simulink model "BD_PAR_AUTO_base_model"  (Simulink 10.3)
settings: Solver=ode1  StartTime=0.0  StopTime=max(cyc_mph(:,1))  FixedStep=1  MaxStep=1  RelTol=1e-3  AbsTol=1e-3
undefined symbols (not defined in the file): acc_dcdc_eff, acc_elec_eff, acc_elec_pwr, acc_mech_eff, acc_mech_pwr, acc_mech_trq, air_cp, amb_tmp, cs_charge_deplete_bool, cs_charge_trq, cs_electric_decel_spd, cs_electric_launch_spd_hi, cs_electric_launch_spd_lo, cs_hi_soc, cs_lo_soc, cs_min_trq_frac, cs_off_trq_frac, cyc_avg_time, cyc_cargo_mass, cyc_elevation_init, cyc_filter_bool, cyc_grade, cyc_mph, enable_sim_stop_distance, enable_sim_stop_max_spd, enable_sim_stop_speed, enable_sim_stop_time, enable_stop, enable_stop_fc, ess_cap_scale, ess_coulombic_eff, ess_init_soc, ess_max_ah_cap, ess_max_volts, ess_min_volts, ess_mod_airflow, ess_mod_cp, ess_mod_init_tmp, ess_module_mass, ess_module_num, ess_on, ess_r_chg, ess_r_dis, ess_res_scale_coef, ess_res_scale_fun, ess_set_tmp, ess_soc, ess_th_calc, ess_th_res_off, ess_th_res_on, ess_tmp, ess_voc, ex_calc, ex_cat_co_frac, ex_cat_ext_cp, ex_cat_ext_emisv, ex_cat_ext_init_tmp, ex_cat_ext_mass, ex_cat_ext_sarea, ex_cat_hc_frac ... (+168)
(part 2 of 15)

== system BD_PAR_AUTO_base_model/hydraulic torque converter for  parallel hybrid <htc> ==
  "req'd output trq and spd (Nm), (rad/s)" : Inport
  "trq and spd available at input (Nm), (rad/s)" : Inport  Port=2
  ">0 " : Saturate  UpperLimit=inf  LowerLimit=0
  >0. : Saturate  UpperLimit=inf  LowerLimit=0
  Block NOTES : Subsystem
      mask Display: disp('Block\nNOTES')
  Constant : Constant  Value=0
  Demux2 : Demux  Outputs=2
  Demux3 : Demux  Outputs=2
  Mux1 : Mux  Inputs=2
  Mux3 : Mux  Inputs=2
  Mux4 : Mux  Inputs=2
  SR : Subsystem
  "T, shifting" : Subsystem
  TR : Subsystem
  Tin= Tout,req/TR : Product  Inputs=/*  SaturateOnIntegerOverflow=on
  To Workspace : ToWorkspace  VariableName=htc_trq_in_r  SampleTime=-1
  To Workspace1 : ToWorkspace  VariableName=htc_spd_in_r  SampleTime=-1
  To Workspace10 : ToWorkspace  VariableName=htc_trq_inertia  SampleTime=-1
  To Workspace2 : ToWorkspace  VariableName=htc_trq_out_r  SampleTime=-1
  To Workspace3 : ToWorkspace  VariableName=htc_spd_out_r  SampleTime=-1
  To Workspace4 : ToWorkspace  VariableName=htc_trq_in_a  SampleTime=-1
  To Workspace5 : ToWorkspace  VariableName=htc_spd_in_a  SampleTime=-1
  To Workspace6 : ToWorkspace  VariableName=htc_trq_out_a  SampleTime=-1
  To Workspace7 : ToWorkspace  VariableName=htc_spd_out_a  SampleTime=-1
  To Workspace8 : ToWorkspace  VariableName=htc_sr_hist  SampleTime=-1
  To Workspace9 : ToWorkspace  VariableName=htc_tr_hist  SampleTime=-1
  Tout= Tin*TR : Product  Inputs=**  SaturateOnIntegerOverflow=on
  Tout_a =  Tout- Tinertia : Sum  Inputs=-+  SaturateOnIntegerOverflow=on
  "Treq, in =  Tin+ Tinertia" : Sum  SaturateOnIntegerOverflow=on
  effect of inertia (Nm) : Subsystem
  "shifting, ignore inertia torque in request" : Switch  Threshold=eps
  win= wout/SR : Product  Inputs=*/  SaturateOnIntegerOverflow=on
  wout= win*SR : Product  Inputs=**  SaturateOnIntegerOverflow=on
  "req'd input trq and spd (Nm), (rad/s)" : Outport  InitialOutput=0
  "trq and spd available at output (Nm), (rad/s)" : Outport  Port=2  InitialOutput=0
  wires:
  [shifting] -> "shifting, ignore inertia torque in request"/2
  >0./1 -> Mux3/2, To Workspace7/1
  wout= win*SR/1 -> >0./1
  Demux3/1 -> To Workspace4/1, Tout= Tin*TR/2
  "trq and spd available at input (Nm), (rad/s)"/1 -> Demux3/1
  Tout= Tin*TR/1 -> Tout_a =  Tout- Tinertia/2
  Mux3/1 -> "trq and spd available at output (Nm), (rad/s)"/1
  win= wout/SR/1 -> ">0 "/1
  "T, shifting"/1(T req) -> Mux4/1, Tin= Tout,req/TR/2, To Workspace2/1
  Demux2/1 -> "T, shifting"/3(Req'd output trq)
  Demux3/2 -> To Workspace5/1, wout= win*SR/2, SR/2(w in), "T, shifting"/4(htc_spd_in_a)
  Mux4/1 -> SR/1(T,w req out)
  SR/1(SR) -> win= wout/SR/2, wout= win*SR/1, To Workspace8/1, "T, shifting"/5(SR), TR/1(SR)
  Tout_a =  Tout- Tinertia/1 -> Mux3/1, To Workspace6/1
  Demux2/2 -> Mux4/2, win= wout/SR/1, effect of inertia (Nm)/1(turbine/output speed (rad/s)), To Workspace3/1
  ">0 "/1 -> To Workspace1/1, Mux1/2
  Constant/1 -> "shifting, ignore inertia torque in request"/1
  effect of inertia (Nm)/1(inertia torque (Nm)) -> Tout_a =  Tout- Tinertia/1, To Workspace10/1, "shifting, ignore inertia torque in request"/3
  TR/1(TR) -> Tout= Tin*TR/1, To Workspace9/1, Tin= Tout,req/TR/1, "T, shifting"/1(TR)
  SR/2(coasting) -> TR/2(coasting)
  Mux1/1 -> "req'd input trq and spd (Nm), (rad/s)"/1
  "Treq, in =  Tin+ Tinertia"/1 -> Mux1/1, To Workspace/1, "T, shifting"/2(Req'd  input trq)
  "shifting, ignore inertia torque in request"/1 -> "Treq, in =  Tin+ Tinertia"/2
  Tin= Tout,req/TR/1 -> "Treq, in =  Tin+ Tinertia"/1
  "req'd output trq and spd (Nm), (rad/s)"/1 -> Demux2/1

== system BD_PAR_AUTO_base_model/mechanical accessory loads <acc> ==
  note: from <fc>
  note: from <fc>
  note: torque req
  note: speed req
  note: aux spd req
  note: torque achieved
  note: speed achieved
  note: aux spd achieved
  note: from <vc>
  In1 : Inport
  In2 : Inport  Port=2
  Constant : Constant  Value=eps
  Demux : Demux  Outputs=2
      settings: DisplayOption=none
  Demux1 : Demux  Outputs=2
      settings: DisplayOption=none
  Logical Operator : Logic
  Mechanical Accessory Loads v2 <acc> : Subsystem  mask{load_on=not(ess_on)*1, acc_max_spd=inf, acc_min_spd=vc_idle_spd+eps, ic_mech_trq=0, ic_mech_pwr=0}
      mask prompts: load_on "Electrical Load Status: 1 on; 0 off"; acc_max_spd "maximum shaft speed for aux. (rad/s)"; acc_min_spd "minimum shaft speed for aux. (rad/s)"; ic_mech_trq "Initial Mechanical Torque of the Accessory Loads (Nm)"; ic_mech_pwr "Initial Mechanical Auxiliary Load Power (W)"
      mask Display: image(imread('bdi_acc_pic.bmp'))
  Mux : Mux  Inputs=3
  Mux1 : Mux  Inputs=3
  Relational Operator : RelationalOperator  Operator=>  RndMeth=Nearest  InputSameDT=on
  Out1 : Outport
  Out2 : Outport  Port=2
  wires:
  [signal_one] -> Mechanical Accessory Loads v2 <acc>/1("requested shaft T and w, out to the driveline  (Nm ; rad/s; rad/s)")
  Mechanical Accessory Loads v2 <acc>/1("requested shaft and belt T and w, in from the prime mover (Nm ; rad/s)") -> Out1/1
  Mechanical Accessory Loads v2 <acc>/2("achieved shaft T and w, out to the driveline (Nm ; rad/s)") -> Out2/1
  [signal_two] -> Mechanical Accessory Loads v2 <acc>/2("achieved shaft and belt T and w, in from the prime mover (Nm ; rad/s)")
  [acc_on] -> Mechanical Accessory Loads v2 <acc>/3(accessory on/off)
  Mux/1 -> [signal_one]
  In1/1 -> Demux/1
  Demux/1 -> Mux/1
  Demux/2 -> Mux/2
  [fc_spd_est] -> Mux/3
  Mux1/1 -> [signal_two]
  In2/1 -> Demux1/1
  Demux1/1 -> Mux1/1
  Demux1/2 -> Mux1/2
  [fc_spd_est] -> Mux1/3
  [fc_spd_est] -> Relational Operator/1
  Constant/1 -> Relational Operator/2
  [engine_on] -> Logical Operator/1
  Relational Operator/1 -> Logical Operator/2
  Logical Operator/1 -> [acc_on]

== system BD_PAR_AUTO_base_model/motor/ controller <mc> par ==
  "torque and speed  req'd at rotor (Nm), (rad/s)" : Inport
  available motor input power (W) : Inport  Port=2
  Block NOTES : Subsystem
      mask Display: disp('Block\nNOTES')
  Constant : Constant  Value=mc_eff_scale
  Demux : Demux  Outputs=2
  Fcn : Fcn  Expr=u[3]-u[1]*u[2]
  Mux2 : Mux  Inputs=2
  Mux3 : Mux  Inputs=3
  N-m drive torque per W input : Subsystem
  Product : Product  SaturateOnIntegerOverflow=on
  Product1 : Product  Inputs=*/  SaturateOnIntegerOverflow=on
  Saturation : Saturate  UpperLimit=max(mc_map_spd)*mc_spd_scale  LowerLimit=0
  Sum : Sum  SaturateOnIntegerOverflow=on
  Sum1 : Sum  Inputs=-+  SaturateOnIntegerOverflow=on
  Switch : Switch
  To WS1 : ToWorkspace  VariableName=mc_pwr_loss
      settings: MaxDataPoints=50000
  To WS2 : ToWorkspace  VariableName=mc_tmp
      settings: MaxDataPoints=50000
  To WS4 : ToWorkspace  VariableName=mc_clt_th_pwr
      settings: MaxDataPoints=50000
  To Workspace10 : ToWorkspace  VariableName=mc_ni_trq_out_a  SampleTime=-1
  To Workspace4 : ToWorkspace  VariableName=mc_trq_out_r  SampleTime=-1
  To Workspace5 : ToWorkspace  VariableName=mc_spd_out_r  SampleTime=-1
  To Workspace8 : ToWorkspace  VariableName=mc_pwr_in_a  SampleTime=-1
  To Workspace9 : ToWorkspace  VariableName=mc_pwr_in_r  SampleTime=-1
  do ex calcs? : Constant  Value=mc_th_calc
  documentation10 : Subsystem
      settings: OpenFcn=web(['file:\\\' which('motor_controller.htm')]);
      mask Display: image(imread('doc_man.jpg'))
  effect of inertia (Nm) : Subsystem
  enforce torque limit : Subsystem
  mc tmp : Subsystem  TreatAsAtomicUnit=on
  motor controller logic interface : Subsystem
  motor speed estimator : Subsystem
  motor/controller input power map (W) : Lookup2D  RowIndex=mc_map_spd*mc_spd_scale  ColumnIndex=mc_map_trq*mc_trq_scale  Table=mc_inpwr_map*mc_spd_scale*mc_trq_scale
  rotor drive torque available (Nm) : Subsystem
  req'd motor input power (W) : Outport  InitialOutput=0
  "drive torque and speed avail. at rotor (Nm), (rad/s)" : Outport  Port=2  InitialOutput=0
  tag scope: mc_spd_out_a=global, mc_trq_out_a=global
  wires:
  motor/controller input power map (W)/1 -> Product/1, Switch/2, Product1/1
  Product/1 -> Switch/3
  Product1/1 -> Switch/1
  Switch/1 -> N-m drive torque per W input/1(req'd input power (W)), motor controller logic interface/2(P_mc_in_1lim)
  Constant/1 -> Product/2, Product1/2
  motor speed estimator/1(Out1) -> motor/controller input power map (W)/1, enforce torque limit/2(limited motor speed (rad/s))
  Saturation/1 -> effect of inertia (Nm)/1(mc_spd_out_a), motor speed estimator/1(mc_spd_out_a), Mux3/2, Mux2/2, [mc_spd_out_a]
  Sum1/1 -> Mux3/1, Mux2/1, [mc_trq_out_a]
  N-m drive torque per W input/1(Nm per W) -> rotor drive torque available (Nm)/1(torque per unit input power (N-m/W))
  Sum/1 -> enforce torque limit/1(req'd motor torque (Nm))
  effect of inertia (Nm)/1(out_1) -> Sum/2, Sum1/1
  enforce torque limit/1(limited motor torque (Nm)) -> N-m drive torque per W input/2(req'd rotor drive torque (Nm)), motor/controller input power map (W)/2
  motor controller logic interface/1(P_mc_in_r) -> To Workspace9/1, req'd motor input power (W)/1
  Mux2/1 -> "drive torque and speed avail. at rotor (Nm), (rad/s)"/1
  Mux3/1 -> Fcn/1
  Fcn/1 -> To WS1/1, mc tmp/1(Qmc_gen)
  do ex calcs?/1 -> mc tmp/Enable
  mc tmp/1(Tmc) -> To WS2/1
  mc tmp/2(Qmc_clt) -> To WS4/1
  [v_prev] -> mc tmp/2(veh spd)
  [key_on] -> mc tmp/3(key ON?)
  Demux/2 -> Saturation/1, To Workspace5/1, motor controller logic interface/1(w_mc_out_r)
  available motor input power (W)/1 -> Mux3/3, To Workspace8/1, rotor drive torque available (Nm)/2(available input power (W))
  Demux/1 -> Sum/1, To Workspace4/1
  "torque and speed  req'd at rotor (Nm), (rad/s)"/1 -> Demux/1
  rotor drive torque available (Nm)/1(rotor drive torque available) -> Sum1/2, To Workspace10/1

== system BD_PAR_AUTO_base_model/power bus <pb> ==
  req'd power output (W) : Inport
  power available from generator (W) : Inport  Port=2
  power available from energy storage (W) : Inport  Port=3
  Abs : Abs
  Abs1 : Abs
  Block NOTES : Subsystem
      mask Display: disp('Block\nNOTES')
  Constant : Constant  Value=1e-9
  Constant1 : Constant  Value=1e-11
  Constant2 : Constant  Value=0
  Constant7 : Constant  Value=ess_on
  Constant8 : Constant  Value=0
  Relational Operator : RelationalOperator  Operator=<=  RndMeth=Nearest  InputSameDT=on
  Relational Operator1 : RelationalOperator  Operator=<=  RndMeth=Nearest  InputSameDT=on
  Sum1 : Sum  Inputs=+-  SaturateOnIntegerOverflow=on
  Sum2 : Sum  SaturateOnIntegerOverflow=on
  Switch : Switch  Threshold=eps
  Switch1 : Switch  Threshold=eps
  To Workspace8 : ToWorkspace  VariableName=pb_pwr_out_a  SampleTime=-1
  To Workspace9 : ToWorkspace  VariableName=pb_pwr_out_r  SampleTime=-1
  not(and(u1,u2)) : Logic  Operator=NAND
  power req'd from generator (W) : Outport
  power req'd from energy storage (W) : Outport  Port=2
  output power  available at bus : Outport  Port=3
  wires:
  power available from energy storage (W)/1 -> Sum2/2
  Constant8/1 -> Switch1/3
  Constant7/1 -> Switch1/2
  Switch1/1 -> power req'd from energy storage (W)/1
  Sum1/1 -> Switch1/1
  Constant/1 -> Relational Operator/2
  Abs/1 -> Relational Operator/1
  Sum2/1 -> Switch/1, Abs/1
  Switch/1 -> output power  available at bus/1, To Workspace8/1
  Constant1/1 -> Relational Operator1/2
  Abs1/1 -> Relational Operator1/1
  Relational Operator1/1 -> not(and(u1,u2))/2
  not(and(u1,u2))/1 -> Switch/2
  Constant2/1 -> Switch/3
  Relational Operator/1 -> not(and(u1,u2))/1
  power available from generator (W)/1 -> Sum1/2, Sum2/1
  req'd power output (W)/1 -> power req'd from generator (W)/1, Sum1/1, To Workspace9/1, Abs1/1

== system BD_PAR_AUTO_base_model/torque coupler <tc> ==
  "torque and speed req'd at output side of torque coupler (Nm), (rad/s)" : Inport
  "torque and speed avail. at main input (Nm), (rad/s)" : Inport  Port=2
  "torque and speed avail. at motor input to tc (Nm), (rad/s)" : Inport  Port=3
  Block NOTES : Subsystem
      mask Display: disp('Block\nNOTES')
  Demux : Demux  Outputs=2
  Demux1 : Demux  Outputs=2
  Demux2 : Demux  Outputs=2
  MinMax : MinMax  Inputs=2
  MinMax1 : MinMax  Inputs=2
  Mux : Mux  Inputs=2
  Mux1 : Mux  Inputs=2
  Mux2 : Mux  Inputs=2
  Product : Product  Inputs=1  SaturateOnIntegerOverflow=on
  Product1 : Product  Inputs=1  SaturateOnIntegerOverflow=on
  To Workspace2 : ToWorkspace  VariableName=tc_trq_out_r  SampleTime=-1
  To Workspace3 : ToWorkspace  VariableName=tc_spd_out_r  SampleTime=-1
  To Workspace4 : ToWorkspace  VariableName=tc_trq_out_a  SampleTime=-1
  To Workspace5 : ToWorkspace  VariableName=tc_spd_out_a  SampleTime=-1
  To Workspace6 : ToWorkspace  VariableName=tc_pwr_in_a  SampleTime=-1
  effect of motor torque at output of tc (Nm) : Gain  Gain=tc_mc_to_fc_ratio  SaturateOnIntegerOverflow=on
  help : Subsystem
      settings: OpenFcn=web(['file:\\\' which('torque_coupler.htm')]);
      mask Display: image(imread('doc_man.jpg'))
  loss (Nm) : Subsystem
  speed of output gear corresponding to motor spd (rad/s) : Gain  Gain=1/tc_mc_to_fc_ratio  SaturateOnIntegerOverflow=on
  speed req'd of motor (rad/s) : Gain  Gain=tc_mc_to_fc_ratio  SaturateOnIntegerOverflow=on
  "sum " : Sum  SaturateOnIntegerOverflow=on
  torque avail. at output side of tc (Nm) : Sum  Inputs=-++  SaturateOnIntegerOverflow=on
  total torque req'd at output gear (Nm) : Sum  SaturateOnIntegerOverflow=on
  total torque req'd of motor (Nm) : Gain  Gain=1/tc_mc_to_fc_ratio  SaturateOnIntegerOverflow=on
  unmet torque request (Nm) : Sum  Inputs=+-  SaturateOnIntegerOverflow=on
  "torque and speed req'd at main input to torque coupler (Nm), (rad/s)" : Outport  InitialOutput=0
  "torque and speed req'd at motor input to torque coupler (Nm), (rad/s)" : Outport  Port=2  InitialOutput=0
  "torque and speed avail. at output side of torque coupler (Nm), (rad/s)" : Outport  Port=3  InitialOutput=0
  wires:
  Product1/1 -> "sum "/2
  "torque and speed avail. at motor input to tc (Nm), (rad/s)"/1 -> Product1/1, Demux2/1
  "torque and speed avail. at main input (Nm), (rad/s)"/1 -> Product/1, Demux1/1
  Product/1 -> "sum "/1
  "sum "/1 -> To Workspace6/1
  Mux/1 -> "torque and speed req'd at main input to torque coupler (Nm), (rad/s)"/1
  "torque and speed req'd at output side of torque coupler (Nm), (rad/s)"/1 -> Demux/1
  Demux/2 -> loss (Nm)/1(tc output speed (rad/s)), Mux/2, MinMax/1, To Workspace3/1
  total torque req'd at output gear (Nm)/1 -> Mux/1, unmet torque request (Nm)/1
  unmet torque request (Nm)/1 -> total torque req'd of motor (Nm)/1
  Demux1/2 -> MinMax/2
  Mux1/1 -> "torque and speed req'd at motor input to torque coupler (Nm), (rad/s)"/1
  total torque req'd of motor (Nm)/1 -> Mux1/1
  speed req'd of motor (rad/s)/1 -> Mux1/2
  loss (Nm)/1(drag torque (Nm)) -> total torque req'd at output gear (Nm)/2, torque avail. at output side of tc (Nm)/1
  Demux1/1 -> unmet torque request (Nm)/2, torque avail. at output side of tc (Nm)/2
  Demux2/1 -> effect of motor torque at output of tc (Nm)/1
  effect of motor torque at output of tc (Nm)/1 -> torque avail. at output side of tc (Nm)/3
  Mux2/1 -> "torque and speed avail. at output side of torque coupler (Nm), (rad/s)"/1
  Demux2/2 -> speed of output gear corresponding to motor spd (rad/s)/1
  speed of output gear corresponding to motor spd (rad/s)/1 -> MinMax1/2
  MinMax/1 -> speed req'd of motor (rad/s)/1, MinMax1/1
  Demux/1 -> total torque req'd at output gear (Nm)/1, To Workspace2/1
  torque avail. at output side of tc (Nm)/1 -> Mux2/1, To Workspace4/1
  MinMax1/1 -> Mux2/2, To Workspace5/1

== system BD_PAR_AUTO_base_model/vehicle <veh> ==
  vehicle speed req'd at end of time step (m/s) : Inport
  tractive force and linear speed achievable (N) : Inport  Port=2
  "(m/s) -> (mph)1" : Gain  Gain=2.23713646532438  SaturateOnIntegerOverflow=on
  Block NOTES : Subsystem
      mask Display: disp('Block\nNOTES')
  Demux1 : Demux  Outputs=2
  Gain : Gain  Gain=0.5  SaturateOnIntegerOverflow=on
  Memory : Memory  InitialCondition=cyc_mph(1,2)*.447
  Mux : Mux  Inputs=2
  Rolling Resistance Force (N) : ToWorkspace  VariableName=Fr  SampleTime=-1
  Sum : Sum  SaturateOnIntegerOverflow=on
  Sum1 : Sum  Inputs=++++  SaturateOnIntegerOverflow=on
  To Workspace2 : ToWorkspace  VariableName=veh_force_r  SampleTime=-1
  To Workspace3 : ToWorkspace  VariableName=veh_spd_r  SampleTime=-1
  To Workspace4 : ToWorkspace  VariableName=veh_force_a  SampleTime=-1
  To Workspace5 : ToWorkspace  VariableName=veh_spd_a  SampleTime=-1
  force req'd to accelerate (N) : Subsystem
  force req'd to ascend (N) : Subsystem
  force req'd to overcome aerodynamic drag (N) : Subsystem
  help : Subsystem
      settings: OpenFcn=web(['file:\\\' which('vehicle.htm')]);
      mask Display: image(imread('doc_man.jpg'))
  record achieved force outputs : Subsystem
  rolling resistance force : Subsystem  BlockChoice=force req'd to overcome rolling resistance (N)
      settings: AttributesFormatString=%<BlockChoice>  TemplateBlock=lib_vehicle/Submodels/rolling resistance force  MemberBlocks=force req'd to overcome rolling resistance (N),force req'd to overcome rolling resistance (N) j2452
  vehicle speed : Subsystem  BlockChoice=vehicle speed (m/s)
      settings: AttributesFormatString=%<BlockChoice>  TemplateBlock=lib_vehicle/Submodels/vehicle speed  MemberBlocks=vehicle speed (m/s),vehicle speed (m/s) j2452
  "tractive force and speed required of tire and wheel (N), (m/s)" : Outport  InitialOutput=0
  tag scope: mpha=global, v_prev=global
  wires:
  vehicle speed/1(vehicle speed achievable at end of time step (m/s)) -> record achieved force outputs/2(spd), "(m/s) -> (mph)1"/1, Memory/1
  tractive force and linear speed achievable (N)/1 -> vehicle speed/2("available tractive force and linear speed (N), (m/s)"), Demux1/1
  Gain/1 -> rolling resistance force/1(average vehicle speed over time step (m/s)), force req'd to overcome aerodynamic drag (N)/1(average vehicle speed over time step (m/s)), Mux/2, To Workspace3/1, force req'd to ascend (N)/1(average vehicle speed over time step (m/s))
  Sum/1 -> Gain/1
  vehicle speed req'd at end of time step (m/s)/1 -> force req'd to accelerate (N)/1(v(m/s)), Sum/1
  Mux/1 -> "tractive force and speed required of tire and wheel (N), (m/s)"/1
  Sum1/1 -> Mux/1, To Workspace2/1
  Demux1/1 -> To Workspace4/1
  Demux1/2 -> To Workspace5/1
  force req'd to overcome aerodynamic drag (N)/1(D aero(N)) -> Sum1/3
  force req'd to accelerate (N)/1((N)) -> Sum1/4
  Memory/1 -> record achieved force outputs/1(spd_prev), [v_prev], vehicle speed/1(vehicle speed at beginning of time step (m/s)), force req'd to accelerate (N)/2(v prev), Sum/2
  "(m/s) -> (mph)1"/1 -> [mpha]
  force req'd to ascend (N)/1((N)) -> Sum1/2
  rolling resistance force/1(Fr (N)) -> Rolling Resistance Force (N)/1, Sum1/1

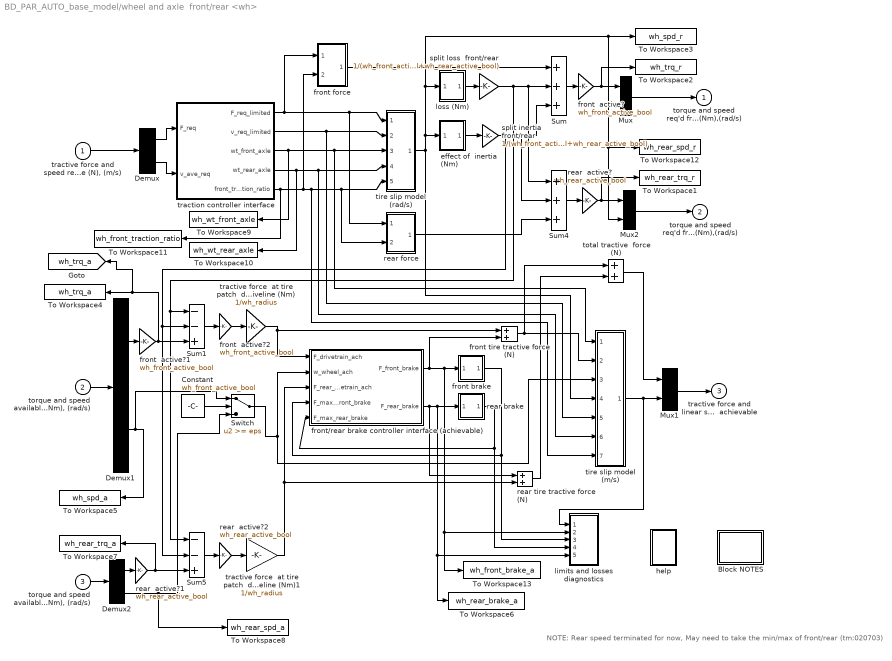
== system BD_PAR_AUTO_base_model/wheel and axle  front/rear <wh> ==
  note: NOTE: Rear speed terminated for now, May need to take the min/max of front/rear (tm:020703)
  "tractive force and speed req'd of tire/road interface (N), (m/s)" : Inport
  "torque and speed available from drivetrain into front axle (Nm), (rad/s)" : Inport  Port=2
  "torque and speed available from drivetrain into rear axle (Nm), (rad/s)" : Inport  Port=3
  Block NOTES : Subsystem
      mask Display: disp('Block\nNOTES')
  Constant : Constant  Value=wh_front_active_bool
  Demux : Demux  Outputs=2
  Demux1 : Demux  Outputs=2
  Demux2 : Demux  Outputs=2
  Mux : Mux  Inputs=2
  Mux1 : Mux  Inputs=2
  Mux2 : Mux  Inputs=2
  Sum : Sum  Inputs=+++  SaturateOnIntegerOverflow=on
  Sum1 : Sum  Inputs=--+  SaturateOnIntegerOverflow=on
  Sum4 : Sum  Inputs=+++  SaturateOnIntegerOverflow=on
  Sum5 : Sum  Inputs=--+  SaturateOnIntegerOverflow=on
  Switch : Switch  Threshold=eps
  To Workspace1 : ToWorkspace  VariableName=wh_rear_trq_r  SampleTime=-1
  To Workspace10 : ToWorkspace  VariableName=wh_wt_rear_axle  SampleTime=-1
  To Workspace11 : ToWorkspace  VariableName=wh_front_traction_ratio  SampleTime=-1
  To Workspace12 : ToWorkspace  VariableName=wh_rear_spd_r  SampleTime=-1
  To Workspace13 : ToWorkspace  VariableName=wh_front_brake_a  SampleTime=-1
  To Workspace2 : ToWorkspace  VariableName=wh_trq_r  SampleTime=-1
  To Workspace3 : ToWorkspace  VariableName=wh_spd_r  SampleTime=-1
  To Workspace4 : ToWorkspace  VariableName=wh_trq_a  SampleTime=-1
  To Workspace5 : ToWorkspace  VariableName=wh_spd_a  SampleTime=-1
  To Workspace6 : ToWorkspace  VariableName=wh_rear_brake_a  SampleTime=-1
  To Workspace7 : ToWorkspace  VariableName=wh_rear_trq_a  SampleTime=-1
  To Workspace8 : ToWorkspace  VariableName=wh_rear_spd_a  SampleTime=-1
  To Workspace9 : ToWorkspace  VariableName=wh_wt_front_axle  SampleTime=-1
  effect of  inertia (Nm) : Subsystem
  front  active? : Gain  Gain=wh_front_active_bool  SaturateOnIntegerOverflow=on
  front  active?1 : Gain  Gain=wh_front_active_bool  SaturateOnIntegerOverflow=on
  front  active?2 : Gain  Gain=wh_front_active_bool  SaturateOnIntegerOverflow=on
  front brake : Subsystem
  front force : Subsystem
  front tire tractive force (N) : Sum  SaturateOnIntegerOverflow=on
  front/rear brake controller interface (achievable) : Subsystem
  help : Subsystem
      settings: OpenFcn=web(['file:\\\' which('advisor_doc.htm')]);
      mask Display: image(imread('doc_man.jpg'))
  limits and losses diagnostics : Subsystem
  loss (Nm) : Subsystem
  rear  active? : Gain  Gain=wh_rear_active_bool  SaturateOnIntegerOverflow=on
  rear  active?1 : Gain  Gain=wh_rear_active_bool  SaturateOnIntegerOverflow=on
  rear  active?2 : Gain  Gain=wh_rear_active_bool  SaturateOnIntegerOverflow=on
  rear brake : Subsystem
  rear force : Subsystem
  rear tire tractive force (N) : Sum  SaturateOnIntegerOverflow=on
  split inertia front/rear : Gain  Gain=1/(wh_front_active_bool+wh_rear_active_bool)  SaturateOnIntegerOverflow=on
  split loss  front/rear : Gain  Gain=1/(wh_front_active_bool+wh_rear_active_bool)  SaturateOnIntegerOverflow=on
  tire slip model (m/s) : Subsystem
  tire slip model (rad/s) : Subsystem
  total tractive  force (N) : Sum  SaturateOnIntegerOverflow=on
  traction controller interface : Subsystem
  tractive force  at tire patch  due to driveline (Nm) : Gain  Gain=1/wh_radius  SaturateOnIntegerOverflow=on
  tractive force  at tire patch  due to driveline (Nm)1 : Gain  Gain=1/wh_radius  SaturateOnIntegerOverflow=on
  torque and speed req'd from drivetrain into front axle (Nm),(rad/s) : Outport  InitialOutput=0
  torque and speed req'd from drivetrain into rear axle (Nm),(rad/s) : Outport  Port=2  InitialOutput=0
  tractive force and linear speed  achievable : Outport  Port=3  InitialOutput=0
  tag scope: wh_trq_a=global
  wires:
  Demux1/2 -> To Workspace5/1, Switch/1
  Constant/1 -> Switch/2
  front  active?2/1 -> tractive force  at tire patch  due to driveline (Nm)/1
  rear  active?2/1 -> tractive force  at tire patch  due to driveline (Nm)1/1
  rear  active?1/1 -> Sum5/3, To Workspace7/1
  front  active?1/1 -> Sum1/3, [wh_trq_a], To Workspace4/1
  rear  active?/1 -> Mux2/1, To Workspace1/1
  front  active?/1 -> To Workspace2/1, Mux/1
  Demux2/2 -> Switch/3, To Workspace8/1
  Demux2/1 -> rear  active?1/1
  rear tire tractive force (N)/1 -> total tractive  force (N)/2
  tractive force  at tire patch  due to driveline (Nm)1/1 -> rear tire tractive force (N)/2, front/rear brake controller interface (achievable)/3(F_rear_drivetrain_ach)
  "torque and speed available from drivetrain into rear axle (Nm), (rad/s)"/1 -> Demux2/1
  Sum5/1 -> rear  active?2/1
  traction controller interface/4(wt_rear_axle) -> To Workspace10/1, tire slip model (m/s)/6(weight borne by  rear axle (N)), tire slip model (rad/s)/4(weight borne by  rear axle (N)1)
  split inertia front/rear/1 -> Sum5/2, Sum1/2, Sum4/2, Sum/3
  split loss  front/rear/1 -> Sum5/1, Sum1/1, Sum4/1, Sum/2
  Mux2/1 -> torque and speed req'd from drivetrain into rear axle (Nm),(rad/s)/1
  Sum4/1 -> rear  active?/1
  rear force/1(Out1) -> Sum4/3
  traction controller interface/5(front_traction_ratio) -> To Workspace11/1, front force/2(In2), rear force/2(In2), tire slip model (rad/s)/5(front traction ratio), tire slip model (m/s)/7(front fraction)
  Demux/1 -> traction controller interface/1(F_req)
  front/rear brake controller interface (achievable)/2(F_rear_brake) -> To Workspace6/1, limits and losses diagnostics/5(rear brake), rear brake/1(F_brake), rear tire tractive force (N)/1
  traction controller interface/1(F_req_limited) -> front force/1(In1), tire slip model (rad/s)/1(total tractive  force requested (N)), rear force/1(In1)
  Switch/1 -> tire slip model (m/s)/3(axle speed available (rad/s)), front/rear brake controller interface (achievable)/2(w_wheel_ach)
  Demux1/1 -> front  active?1/1
  Sum/1 -> front  active?/1
  Mux/1 -> torque and speed req'd from drivetrain into front axle (Nm),(rad/s)/1
  traction controller interface/3(wt_front_axle) -> To Workspace9/1, tire slip model (m/s)/1(weight borne  by front axle (N)), tire slip model (rad/s)/3(weight borne by front axle (N))
  rear brake/1(F_brake_max) -> limits and losses diagnostics/4(rear brake max), front/rear brake controller interface (achievable)/5(F_max_rear_brake)
  front brake/1(F_brake_max) -> limits and losses diagnostics/3(front brake max), front/rear brake controller interface (achievable)/4(F_max_front_brake)
  front tire tractive force (N)/1 -> total tractive  force (N)/1, tire slip model (m/s)/2(total tractive  force available (N))
  front/rear brake controller interface (achievable)/1(F_front_brake) -> To Workspace13/1, limits and losses diagnostics/2(front brake), front brake/1(F_brake), front tire tractive force (N)/2
  "torque and speed available from drivetrain into front axle (Nm), (rad/s)"/1 -> Demux1/1
  total tractive  force (N)/1 -> Mux1/1
  Mux1/1 -> tractive force and linear speed  achievable/1
  front force/1(Out1) -> Sum/1
  tire slip model (rad/s)/1(slip-augmented rotational speed (rad/s)) -> tire slip model (m/s)/4(axle speed req'd (rad/s)), To Workspace12/1, Mux2/2, Mux/2, To Workspace3/1, loss (Nm)/1(axle speed (rad/s)), effect of  inertia (Nm)/1(axle input speed (rad/s))
  "tractive force and speed req'd of tire/road interface (N), (m/s)"/1 -> Demux/1
  loss (Nm)/1(drag torque (Nm)) -> split loss  front/rear/1
  effect of  inertia (Nm)/1(inertia torque (Nm)) -> split inertia front/rear/1
  Sum1/1 -> front  active?2/1
  tractive force  at tire patch  due to driveline (Nm)/1 -> front tire tractive force (N)/1, front/rear brake controller interface (achievable)/1(F_drivetrain_ach)
  tire slip model (m/s)/1(possible vehicle speed (m/s)) -> limits and losses diagnostics/1(speed), Mux1/2
  Demux/2 -> traction controller interface/2(v_ave_req)
  traction controller interface/2(v_req_limited) -> tire slip model (m/s)/5(vehicle speed required (m/s)), tire slip model (rad/s)/2(requested time-step average vehicle speed (m/s))

== system BD_PAR_AUTO_base_model/<vc> par auto/braking strategy ==
  req'd speed (m/s) : Inport
  slip-limited force req'd (N) : Inport  Port=2
  Block NOTES : Subsystem
      mask Display: disp('Block\nNOTES')
  Constant : Constant  Value=0
  Constant1 : Constant
  Constant2 : Constant  Value=0
  Keep frac>0 : Saturate  UpperLimit=1  LowerLimit=0
  Product : Product  InputSameDT=on  RndMeth=Zero  SaturateOnIntegerOverflow=on  OutDataTypeStr=Inherit: Same as first input
  Product1 : Product  InputSameDT=on  RndMeth=Zero  SaturateOnIntegerOverflow=on  OutDataTypeStr=Inherit: Same as first input
  Sum : Sum  Inputs=--+  InputSameDT=on  SaturateOnIntegerOverflow=on  OutDataTypeStr=Inherit: Same as first input
  Switch : Switch
  Switch1 : Switch
  convert (mph) : Gain  Gain=2.2371  SaturateOnIntegerOverflow=on  OutDataTypeStr=Inherit: Same as input  ParamDataTypeStr=Inherit: Same as input
  front driveline braking fraction : Lookup  InputValues=wh_fa_dl_brake_mph  Table=wh_fa_dl_brake_frac
  front friction braking fraction : Lookup  InputValues=wh_fa_fric_brake_mph  Table=wh_fa_fric_brake_frac
  req'd front brake force (N) : Outport  InitialOutput=0
  req'd rear brake force (N) : Outport  Port=2  InitialOutput=0
  wires:
  Constant1/1 -> Sum/3
  front friction braking fraction/1 -> Sum/1, Product/2
  front driveline braking fraction/1 -> Sum/2
  convert (mph)/1 -> front driveline braking fraction/1, front friction braking fraction/1
  req'd speed (m/s)/1 -> convert (mph)/1
  Switch1/1 -> req'd rear brake force (N)/1
  Constant2/1 -> Switch1/1
  Product1/1 -> Switch1/3
  Switch/1 -> req'd front brake force (N)/1
  slip-limited force req'd (N)/1 -> Switch1/2, Product1/1, Product/1, Switch/2
  Product/1 -> Switch/3
  Constant/1 -> Switch/1
  Sum/1 -> Keep frac>0/1
  Keep frac>0/1 -> Product1/2

== system BD_PAR_AUTO_base_model/<vc> par auto/config traction control ==
  time-average vehicle speed  req'd (m/s) : Inport
  vehicle speed at beginning of time  step (m/s) : Inport  Port=2
  total tractive force req'd (N) : Inport  Port=3
  traction control 2 axle : Subsystem
  req'd force (N) : Outport
  req'd speed (m/s) : Outport  Port=2
  weight on front axle (N) : Outport  Port=3
  weight on rear axle (N) : Outport  Port=4
  front/total  traction ratio : Outport  Port=5
  wires:
  time-average vehicle speed  req'd (m/s)/1 -> traction control 2 axle/1(time-average vehicle speed  req'd (m/s))
  vehicle speed at beginning of time  step (m/s)/1 -> traction control 2 axle/2(vehicle speed at beginning of time  step (m/s))
  total tractive force req'd (N)/1 -> traction control 2 axle/3(total tractive force req'd (N))
  traction control 2 axle/1(req'd force (N)) -> req'd force (N)/1
  traction control 2 axle/2(req'd speed (m/s)) -> req'd speed (m/s)/1
  traction control 2 axle/3(weight on front axle (N)) -> weight on front axle (N)/1
  traction control 2 axle/4(weight on rear axle (N)) -> weight on rear axle (N)/1
  traction control 2 axle/5(front/total  traction ratio) -> front/total  traction ratio/1

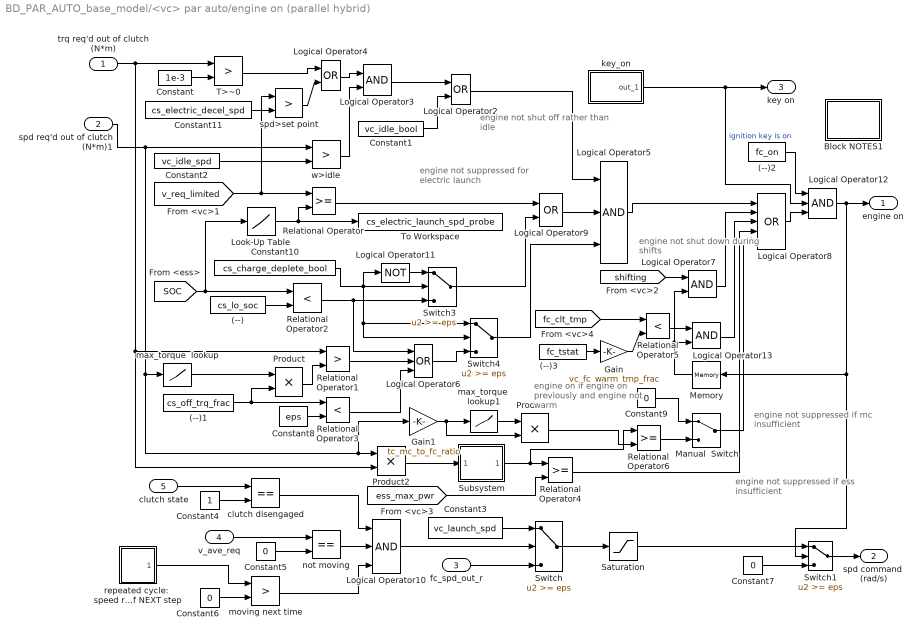
== system BD_PAR_AUTO_base_model/<vc> par auto/engine on (parallel hybrid) ==
  note: engine not suppressed
      | if mc insufficient
  note: engine not shut
      | down during shifts
  note: engine on if engine on
      | previously and engine
      | not warm
  note: engine not shut off
      |  rather than idle
  note: engine not
      | suppressed for
      | electric launch
  note: engine not suppressed if
      | ess insufficient
  trq req'd out of clutch (N*m) : Inport
  spd req'd out of clutch (N*m)1 : Inport  Port=2
  fc_spd_out_r : Inport  Port=3
  v_ave_req : Inport  Port=4
  clutch state : Inport  Port=5
  (--) : Constant  Value=cs_lo_soc
  (--)1 : Constant  Value=cs_off_trq_frac
  (--)2 : Constant  Value=fc_on
  (--)3 : Constant  Value=fc_tstat
  Block NOTES1 : Subsystem
      mask Display: disp('Block\nNOTES')
  Constant : Constant  Value=1e-3
  Constant1 : Constant  Value=vc_idle_bool
  Constant10 : Constant  Value=cs_charge_deplete_bool
  Constant11 : Constant  Value=cs_electric_decel_spd
  Constant2 : Constant  Value=vc_idle_spd
  Constant3 : Constant  Value=vc_launch_spd
  Constant4 : Constant
  Constant{5..7,9} (4 alike) : Constant  Value=0
  Constant8 : Constant  Value=eps
  Gain : Gain  Gain=vc_fc_warm_tmp_frac  SaturateOnIntegerOverflow=on  OutDataTypeStr=Inherit: Same as input  ParamDataTypeStr=Inherit: Same as input
  Gain1 : Gain  Gain=tc_mc_to_fc_ratio  SaturateOnIntegerOverflow=on  OutDataTypeStr=Inherit: Same as input  ParamDataTypeStr=Inherit: Same as input
  Logical Operator10 : Logic  Inputs=3
  Logical Operator11 : Logic  Operator=NOT  Inputs=1
  Logical Operator12 : Logic  Inputs=3
  Logical Operator13 : Logic
  Logical Operator2 : Logic  Operator=OR
  Logical Operator3 : Logic
  Logical Operator4 : Logic  Operator=OR
  Logical Operator5 : Logic  Inputs=3
  Logical Operator6 : Logic  Operator=OR  Inputs=3
  Logical Operator7 : Logic
  Logical Operator8 : Logic  Operator=OR  Inputs=5
  Logical Operator9 : Logic  Operator=OR
  Look-Up Table : Lookup  InputValues=[cs_lo_soc cs_hi_soc cs_hi_soc+eps]  Table=[cs_electric_launch_spd_lo cs_electric_launch_spd_hi cs_electric_launch_spd_hi]
  Manual  Switch : ManualSwitch
  Memory : Memory  InitialCondition=cyc_mph(1,2)>0
  Product : Product  InputSameDT=on  RndMeth=Zero  SaturateOnIntegerOverflow=on  OutDataTypeStr=Inherit: Same as first input
  Product2 : Product  InputSameDT=on  RndMeth=Zero  SaturateOnIntegerOverflow=on  OutDataTypeStr=Inherit: Same as first input
  Product3 : Product  InputSameDT=on  RndMeth=Zero  SaturateOnIntegerOverflow=on  OutDataTypeStr=Inherit: Same as first input
  Relational Operator : RelationalOperator  RndMeth=Nearest  InputSameDT=on
  Relational Operator1 : RelationalOperator  Operator=>  RndMeth=Nearest  InputSameDT=on
  Relational Operator2 : RelationalOperator  Operator=<  RndMeth=Nearest  InputSameDT=on
  Relational Operator3 : RelationalOperator  Operator=<  RndMeth=Nearest  InputSameDT=on
  Relational Operator4 : RelationalOperator  RndMeth=Nearest  InputSameDT=on
  Relational Operator5 : RelationalOperator  Operator=<  RndMeth=Nearest  InputSameDT=on
  Relational Operator6 : RelationalOperator  RndMeth=Nearest  InputSameDT=on
  Saturation : Saturate  UpperLimit=max(fc_map_spd)*fc_spd_scale  LowerLimit=vc_idle_spd*vc_idle_bool
  Subsystem : Subsystem  mask(Running Average){n=3}
      mask prompts: n "Averaging Time Steps (#)"
      mask help: Running Average
      mask Help: Output is the average of the last (Averaging Time) seconds of input.
      mask Display: disp('Running\nAverage')
  Switch{,1,3..4} (4 alike) : Switch  Threshold=eps
  T>~0 : RelationalOperator  Operator=>  RndMeth=Nearest  InputSameDT=on
  To Workspace : ToWorkspace  VariableName=cs_electric_launch_spd_probe  SampleTime=-1
  clutch disengaged : RelationalOperator  Operator===  RndMeth=Nearest  InputSameDT=on
  key_on : Subsystem  mask(Repeating table){t=vc_key_on(:,1), y=vc_key_on(:,2)}
      mask prompts: t "Time values:"; y "Output values:"
      mask help:
      | Repeating table.
      | Enter values of time and output for first cycle.
      mask init:
      | period = max(t);
      mask Help: Repeats cycle given in table. Time values should be monotonically increasing.
  max_torque  lookup : Lookup  InputValues=fc_map_spd*fc_spd_scale  Table=fc_max_trq*fc_trq_scale
  max_torque  lookup1 : Lookup  InputValues=mc_map_spd*mc_spd_scale  Table=mc_max_trq*mc_trq_scale*mc_overtrq_factor
  moving next time : RelationalOperator  Operator=>  RndMeth=Nearest  InputSameDT=on
  not moving : RelationalOperator  Operator===  RndMeth=Nearest  InputSameDT=on
  repeated cycle:  speed required at end of NEXT step : Subsystem  mask(Forward looking repeating table){t=cyc_mph(:,1), y=cyc_mph(:,2)}
      mask prompts: t "Time values:"; y "Output values:"
      mask help:
      | Forward looking repeating table.
      | Enter values of time and output for first cycle.
      mask init:
      | period = max(t);
      mask Help: Repeats cycle given in table with a one time step forward offset. Time values should be monotonically increasing.
  spd>set point : RelationalOperator  Operator=>  RndMeth=Nearest  InputSameDT=on
  w>idle : RelationalOperator  Operator=>  RndMeth=Nearest  InputSameDT=on
  engine on : Outport
  spd command  (rad/s) : Outport  Port=2
  key on : Outport  Port=3
  wires:
  Subsystem/1(out_1) -> Relational Operator6/1, Relational Operator4/1
  Relational Operator6/1 -> Manual  Switch/2
  Manual  Switch/1 -> Logical Operator8/5
  Product3/1 -> Relational Operator6/2
  Constant9/1 -> Manual  Switch/1
  Gain1/1 -> Product3/2, max_torque  lookup1/1
  max_torque  lookup1/1 -> Product3/1
  [v_req_limited] -> spd>set point/1, Relational Operator/1
  Logical Operator4/1 -> Logical Operator3/1
  T>~0/1 -> Logical Operator4/1
  spd>set point/1 -> Logical Operator4/2
  Constant11/1 -> spd>set point/2
  clutch disengaged/1 -> Logical Operator10/1
  Relational Operator4/1 -> Logical Operator8/4
  Product2/1 -> Subsystem/1(in_1)
  [ess_max_pwr] -> Relational Operator4/2
  Constant4/1 -> clutch disengaged/2
  clutch state/1 -> clutch disengaged/1
  Constant5/1 -> not moving/2
  v_ave_req/1 -> not moving/1
  not moving/1 -> Logical Operator10/2
  moving next time/1 -> Logical Operator10/3
  Constant6/1 -> moving next time/2
  repeated cycle:  speed required at end of NEXT step/1(out_1) -> moving next time/1
  Constant7/1 -> Switch1/3
  Switch1/1 -> spd command  (rad/s)/1
  Saturation/1 -> Switch1/1
  fc_spd_out_r/1 -> Switch/3
  Logical Operator10/1 -> Switch/2
  Switch/1 -> Saturation/1
  Constant3/1 -> Switch/1
  (--)/1 -> Relational Operator2/2
  [SOC] -> Look-Up Table/1, Relational Operator2/1
  Logical Operator11/1 -> Switch3/1
  Relational Operator2/1 -> Logical Operator6/1, Switch3/3
  Constant10/1 -> Logical Operator11/1, Switch3/2, Switch4/2, Switch4/1
  Look-Up Table/1 -> To Workspace/1, Relational Operator/2
  Relational Operator/1 -> Logical Operator9/1
  Switch4/1 -> Logical Operator5/3
  Logical Operator9/1 -> Logical Operator5/2
  Logical Operator2/1 -> Logical Operator5/1
  key_on/1(out_1) -> Logical Operator12/2, key on/1  "ignition key is on"
  Logical Operator8/1 -> Logical Operator12/3
  (--)3/1 -> Gain/1
  Gain/1 -> Relational Operator5/2
  Logical Operator13/1 -> Logical Operator8/3
  [fc_clt_tmp] -> Relational Operator5/1
  Relational Operator5/1 -> Logical Operator13/1
  Memory/1 -> Logical Operator13/2, Logical Operator7/2
  Relational Operator1/1 -> Logical Operator6/2
  Logical Operator5/1 -> Logical Operator8/1
  spd req'd out of clutch (N*m)1/1 -> w>idle/1, Gain1/1, Product2/1, max_torque  lookup/1
  w>idle/1 -> Logical Operator3/2
  Logical Operator3/1 -> Logical Operator2/1
  Constant1/1 -> Logical Operator2/2
  trq req'd out of clutch (N*m)/1 -> Relational Operator1/1, Product2/2, T>~0/1
  Logical Operator7/1 -> Logical Operator8/2
  [shifting] -> Logical Operator7/1
  Constant/1 -> T>~0/2
  Constant2/1 -> w>idle/2
  Switch3/1 -> Logical Operator9/2
  Logical Operator6/1 -> Switch4/3
  Relational Operator3/1 -> Logical Operator6/3
  Constant8/1 -> Relational Operator3/2
  (--)1/1 -> Relational Operator3/1, Product/2
  Product/1 -> Relational Operator1/2
  max_torque  lookup/1 -> Product/1
  (--)2/1 -> Logical Operator12/1
  Logical Operator12/1 -> engine on/1, Memory/1, Switch1/2

== system BD_PAR_AUTO_base_model/<vc> par auto/front and rear brake controller (achievable) ==
  total tractive force req'd (N) : Inport
  tractive force available from  front drivetrain (N) : Inport  Port=2
  axle speed possible (rad/s) : Inport  Port=3
  max front brake force (N) : Inport  Port=4
  max rear brake force (N) : Inport  Port=5
  tractive force available from  rear drivetrain (N) : Inport  Port=6
  Block NOTES : Subsystem
      mask Display: disp('Block\nNOTES')
  Constant : Constant  Value=0
  Constant1 : Constant  Value=0
  MinMax : MinMax  Inputs=2  InputSameDT=on  SaturateOnIntegerOverflow=on
  MinMax1 : MinMax  Inputs=2  InputSameDT=on  SaturateOnIntegerOverflow=on
  MinMax2 : MinMax  Function=max  Inputs=2  InputSameDT=on  SaturateOnIntegerOverflow=on
  Sum1 : Sum  Inputs=+--  InputSameDT=on  SaturateOnIntegerOverflow=on  OutDataTypeStr=Inherit: Same as first input
  Sum2 : Sum  Inputs=+-  InputSameDT=on  SaturateOnIntegerOverflow=on  OutDataTypeStr=Inherit: Same as first input
  Switch: braking force to be split between friction brakes (N) : Switch
  braking force supplied by front friction brakes (N) : Subsystem
  "m/s -> mph (mph)" : Gain  Gain=2.237  SaturateOnIntegerOverflow=on  OutDataTypeStr=Inherit: Same as input  ParamDataTypeStr=Inherit: Same as input
  "rad/s -> m/s (m/s)" : Gain  Gain=wh_radius  SaturateOnIntegerOverflow=on  OutDataTypeStr=Inherit: Same as input  ParamDataTypeStr=Inherit: Same as input
  rear braking force req'd (N) : Switch
  front-axle braking force (N) : Outport  InitialOutput=0
  rear-axle braking force (N) : Outport  Port=2  InitialOutput=0
  wires:
  tractive force available from  rear drivetrain (N)/1 -> Sum1/3
  braking force supplied by front friction brakes (N)/1(braking force from front-axle friction brakes (N)) -> front-axle braking force (N)/1, Sum2/2
  Switch: braking force to be split between friction brakes (N)/1 -> Sum2/1, rear braking force req'd (N)/2, braking force supplied by front friction brakes (N)/1(add'l braking force req'd (N))
  "m/s -> mph (mph)"/1 -> braking force supplied by front friction brakes (N)/2(possible speed (mph))
  Constant/1 -> MinMax1/1, Switch: braking force to be split between friction brakes (N)/1
  MinMax1/1 -> Switch: braking force to be split between friction brakes (N)/3
  Sum1/1 -> MinMax1/2
  total tractive force req'd (N)/1 -> Switch: braking force to be split between friction brakes (N)/2, Sum1/1
  tractive force available from  front drivetrain (N)/1 -> Sum1/2
  axle speed possible (rad/s)/1 -> "rad/s -> m/s (m/s)"/1
  "rad/s -> m/s (m/s)"/1 -> "m/s -> mph (mph)"/1
  MinMax2/1 -> rear-axle braking force (N)/1
  rear braking force req'd (N)/1 -> MinMax2/1
  Sum2/1 -> MinMax/2
  MinMax/1 -> rear braking force req'd (N)/3
  Constant1/1 -> MinMax/1, rear braking force req'd (N)/1
  max front brake force (N)/1 -> braking force supplied by front friction brakes (N)/3(max front brake force (N))
  max rear brake force (N)/1 -> MinMax2/2

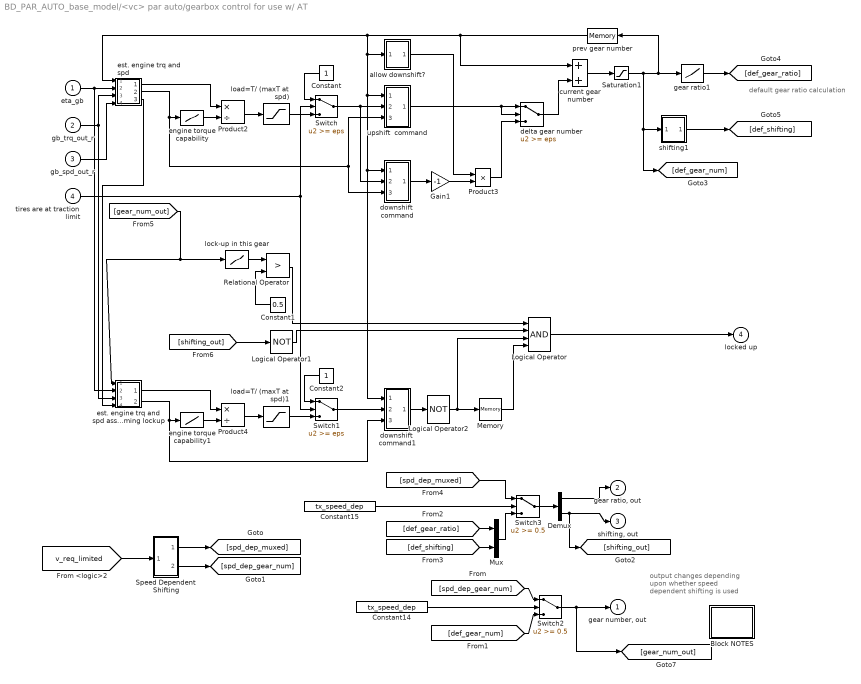
== system BD_PAR_AUTO_base_model/<vc> par auto/gearbox control for use w/ AT ==
  note: output changes depending
      | upon whether speed
      | dependent shifting is used
  note: default gear ratio
      | calculation
  eta_gb : Inport
  gb_trq_out_r : Inport  Port=2
  gb_spd_out_r : Inport  Port=3
  tires are at traction limit : Inport  Port=4
  Block NOTES : Subsystem
      mask Display: disp('Block\nNOTES')
  Constant : Constant
  Constant1 : Constant  Value=0.5
  Constant14 : Constant  Value=tx_speed_dep
  Constant15 : Constant  Value=tx_speed_dep
  Constant2 : Constant
  Demux : Demux  Outputs=2
      settings: DisplayOption=none
  Gain1 : Gain  Gain=-1  SaturateOnIntegerOverflow=on  OutDataTypeStr=Inherit: Same as input  ParamDataTypeStr=Inherit: Same as input
  Logical Operator : Logic  Inputs=4
  Logical Operator1 : Logic  Operator=NOT  Inputs=1
  Logical Operator2 : Logic  Operator=NOT  Inputs=1
  Memory : Memory
  Mux : Mux  Inputs=2
  Product2 : Product  Inputs=*/  InputSameDT=on  RndMeth=Zero  SaturateOnIntegerOverflow=on  OutDataTypeStr=Inherit: Same as first input
  Product3 : Product  InputSameDT=on  RndMeth=Zero  SaturateOnIntegerOverflow=on  OutDataTypeStr=Inherit: Same as first input
  Product4 : Product  Inputs=*/  InputSameDT=on  RndMeth=Zero  SaturateOnIntegerOverflow=on  OutDataTypeStr=Inherit: Same as first input
  Relational Operator : RelationalOperator  Operator=>  RndMeth=Nearest  InputSameDT=on
  Saturation1 : Saturate  UpperLimit=gb_gears_num  LowerLimit=1
  Speed Dependent Shifting : Subsystem
  Switch : Switch  Threshold=eps
  Switch1 : Switch  Threshold=eps
  Switch2 : Switch  Threshold=0.5
  Switch3 : Switch  Threshold=0.5
  allow downshift? : Subsystem
  current gear number : Sum  InputSameDT=on  SaturateOnIntegerOverflow=on  OutDataTypeStr=Inherit: Same as first input
  delta gear number : Switch  Threshold=eps
  downshift  command : Subsystem
  downshift  command1 : Subsystem
  engine torque capability : Lookup  InputValues=fc_map_spd*fc_spd_scale  Table=fc_max_trq*fc_trq_scale+eps
  engine torque capability1 : Lookup  InputValues=fc_map_spd*fc_spd_scale  Table=fc_max_trq*fc_trq_scale+eps
  est. engine trq and spd : Subsystem
  est. engine trq and spd assuming lockup : Subsystem
  gear ratio1 : Lookup  InputValues=[1:length(gb_ratio)]  Table=gb_ratio
  load=T/ (maxT at spd) : Saturate  UpperLimit=1  LowerLimit=-1
  load=T/ (maxT at spd)1 : Saturate  UpperLimit=1  LowerLimit=-1
  lock-up in this gear : Lookup  InputValues=[1:length(htc_lockup)]  Table=htc_lockup
  prev gear number : Memory  InitialCondition=gb_num_init
  shifting1 : Subsystem
  upshift  command : Subsystem
  "gear number, out" : Outport  InitialOutput=0
  "gear ratio, out" : Outport  Port=2  InitialOutput=0
  "shifting, out" : Outport  Port=3  InitialOutput=0
  locked up : Outport  Port=4  InitialOutput=0
  wires:
  [gear_num_out] -> est. engine trq and spd assuming lockup/1(new gear number), lock-up in this gear/1
  Demux/1 -> "gear ratio, out"/1
  Switch2/1 -> [gear_num_out], "gear number, out"/1
  Demux/2 -> [shifting_out], "shifting, out"/1
  Speed Dependent Shifting/2(gear number) -> [spd_dep_gear_num]
  Speed Dependent Shifting/1(gear ratio and shifting) -> [spd_dep_muxed]
  [v_req_limited] -> Speed Dependent Shifting/1("velocity required (limited) ")
  [def_gear_num] -> Switch2/3
  [spd_dep_gear_num] -> Switch2/1
  Constant14/1 -> Switch2/2
  Switch3/1 -> Demux/1
  [def_shifting] -> Mux/2
  [def_gear_ratio] -> Mux/1
  Mux/1 -> Switch3/3
  [spd_dep_muxed] -> Switch3/1
  Constant15/1 -> Switch3/2
  [shifting_out] -> Logical Operator1/1
  lock-up in this gear/1 -> Relational Operator/1
  Constant1/1 -> Relational Operator/2
  shifting1/1(out_1) -> [def_shifting]
  downshift  command1/1(command) -> Logical Operator2/1
  load=T/ (maxT at spd)1/1 -> Switch1/3
  Memory/1 -> Logical Operator/4
  Switch1/1 -> downshift  command1/2(engine load)
  Logical Operator/1 -> locked up/1
  Gain1/1 -> Product3/2
  upshift  command/1(command) -> delta gear number/1, delta gear number/2
  Switch/1 -> upshift  command/2(engine load), downshift  command/2(engine load)
  Logical Operator2/1 -> Memory/1, Logical Operator/3
  est. engine trq and spd assuming lockup/2(est eng spd (rad/s)) -> downshift  command1/3(engine speed), engine torque capability1/1
  est. engine trq and spd/3(gb_spd_in_est (rad/s)1) -> est. engine trq and spd assuming lockup/4(gb_spd_in_est)
  tires are at traction limit/1 -> Switch/2, Switch1/2
  gb_trq_out_r/1 -> est. engine trq and spd assuming lockup/3(gb_trq_out_r), est. engine trq and spd/3(gb_trq_out_r)
  eta_gb/1 -> est. engine trq and spd assuming lockup/2(" prev eta_gb"), est. engine trq and spd/2(" prev eta_gb")
  est. engine trq and spd assuming lockup/1(est eng trq (Nm)) -> Product4/1
  engine torque capability1/1 -> Product4/2
  Product4/1 -> load=T/ (maxT at spd)1/1
  Constant2/1 -> Switch1/1
  Relational Operator/1 -> Logical Operator/1
  Logical Operator1/1 -> Logical Operator/2
  downshift  command/1(command) -> Gain1/1
  load=T/ (maxT at spd)/1 -> Switch/3
  est. engine trq and spd/1(est eng trq (Nm)) -> Product2/1
  engine torque capability/1 -> Product2/2
  current gear number/1 -> Saturation1/1
  Product3/1 -> delta gear number/3
  allow downshift?/1(allow shift) -> Product3/1
  delta gear number/1 -> current gear number/2
  Product2/1 -> load=T/ (maxT at spd)/1
  Constant/1 -> Switch/1
  Saturation1/1 -> [def_gear_num], shifting1/1(gear number), prev gear number/1, gear ratio1/1
  prev gear number/1 -> est. engine trq and spd/1(prev gear number), allow downshift?/1(prev gearnum), downshift  command1/1(prev gear number), downshift  command/1(prev gear number), upshift  command/1(prev gear number), current gear number/1
  gear ratio1/1 -> [def_gear_ratio]
  gb_spd_out_r/1 -> est. engine trq and spd/4(gb_spd_out_r)
  est. engine trq and spd/2(est eng spd (rad/s)) -> engine torque capability/1, upshift  command/3(engine speed), downshift  command/3(engine speed)
